simulink model "read_power_16chan"  (R2013a)
settings: Solver=VariableStepDiscrete  StartTime=0.0  StopTime=10000  RelTol=1e-3
libraries: xbsIndex_r4 x649, casper_library_misc x36, simulink x16, xps_library x1
(part 1 of 7)
settings Model: Creator=root  LastModifiedBy=root

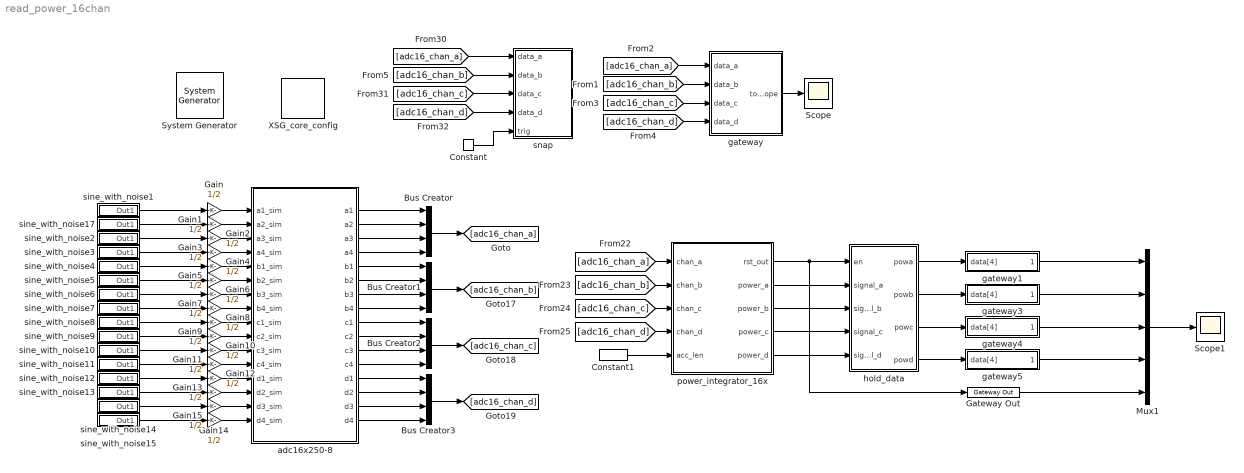
== system read_power_16chan ==
  " System Generator" : xbsIndex_r4/ System Generator  Tag=genX  xilinxfamily=virtex6  part=xc6vsx475t  speed=-1  package=ff1759  synthesis_tool=XST  clock_wrapper=Clock Enables  directory=./read_power_16chan/sysgen  proj_type=Project Navigator  Synth_file=XST Defaults  Impl_file=ISE Defaults  testbench=off  simulink_period=1  sysclk_period=5  dcm_input_clock_period=100  incr_netlist=off  trim_vbits=Everywhere in SubSystem  dbl_ovrd=According to Block Masks  core_generation=According to Block Masks  run_coregen=off  deprecated_control=off  eval_field=0  block_type=sysgen
  Bus Creator{,1..3} (4 alike) : BusCreator
  Constant : xbsIndex_r4/Constant  const=1  gui_display_data_type=Boolean  arith_type=Boolean  n_bits=16  bin_pt=14  preci_type=Single  exp_width=8  frac_width=24  explicit_period=off  period=1  equ=P=C  opselect=C  inp2=PCIN>>17  opr=+  inp1=P  carry=CIN  dbl_ovrd=off  block_type=constant
  Constant1 : xbsIndex_r4/Constant  const=255  gui_display_data_type=Fixed-point  arith_type=Unsigned  n_bits=10  bin_pt=0  preci_type=Single  exp_width=8  frac_width=24  explicit_period=off  period=1  equ=P=C  opselect=C  inp2=PCIN>>17  opr=+  inp1=P  carry=CIN  dbl_ovrd=off  block_type=constant
  Gain{,1..15} (16 alike) : Gain  Gain=1/2
  Gateway Out : xbsIndex_r4/Gateway Out  inherit_from_input=off  hdl_port=on  timing_constraint=None  locs_specified=off  LOCs={}  UseAsDAC=off  DACChannel='1'  block_type=gatewayout
  Mux1 : Mux  Inputs=5
  Scope : Scope
  Scope1 : Scope
  XSG_core_config : xps_library/XSG_core_config  Tag=xps:xsg  hw_sys=ROACH2:sx475t  clk_src=adc0_clk  ROACH_clk_src=sys_clk  ROACH2_clk_src=adc0_clk  MKDIG_clk_src=sys_clk  clk_rate=200  sample_period=1  synthesis_tool=XST
  adc16x250-8 : Subsystem  Tag=xps:adc16  AncestorBlock=xps_library/ADCs/adc16x250-8  mask(ADC16){board_count=1, roach2_rev=2, zdok_rev=2}
      mask prompts: board_count "Number of ADC16 Boards"; roach2_rev "ROACH2 Revision"; zdok_rev "ZDOK Pinout Revision"
      mask help: 16-input ADC. When using one ADC16 board, it must be in ZDOK0.
      mask init:
      | % Only board_count is needed by init function
      | adc16_init(gcb, ...
      |     'board_count', board_count);
      settings: AttributesFormatString=r2 rev%<roach2_rev>\nzdok rev%<zdok_rev>
      mask Help:
      | This is the CASPER "yellow block" for the CASPER ADC16 board.  Each ADC
      | board has four ADC chips.  Each ADC chip accepts four inputs.  The four
      | 8-bit outputs from each ADC chip are concatenated into a 32-bit signal.
      mask TypeOptions board_count: 1 | 2
      mask TypeOptions roach2_rev: 1 | 2
      mask TypeOptions zdok_rev: 1 | 2
  gateway : Subsystem
  gateway1 : Subsystem
  gateway3 : Subsystem
  gateway4 : Subsystem
  gateway5 : Subsystem
  hold_data : Subsystem
  power_integrator_16x : Subsystem
  sine_with_noise1 : Subsystem
  sine_with_noise10 : Subsystem
  sine_with_noise11 : Subsystem
  sine_with_noise12 : Subsystem
  sine_with_noise13 : Subsystem
  sine_with_noise14 : Subsystem
  sine_with_noise15 : Subsystem
  sine_with_noise17 : Subsystem
  sine_with_noise2 : Subsystem
  sine_with_noise3 : Subsystem
  sine_with_noise4 : Subsystem
  sine_with_noise5 : Subsystem
  sine_with_noise6 : Subsystem
  sine_with_noise7 : Subsystem
  sine_with_noise8 : Subsystem
  sine_with_noise9 : Subsystem
  snap : Subsystem
  wires:
  adc16x250-8/3(a3) -> Bus Creator/3
  adc16x250-8/2(a2) -> Bus Creator/2
  adc16x250-8/4(a4) -> Bus Creator/4
  Constant/1 -> snap/5(trig)
  gateway/1(to_scope) -> Scope/1
  adc16x250-8/1(a1) -> Bus Creator/1
  Bus Creator/1 -> [adc16_chan_a]
  power_integrator_16x/2(power_a) -> hold_data/2(signal_a)
  hold_data/1(powa) -> gateway1/1(data[4])
  power_integrator_16x/1(rst_out) -> Gateway Out/1, hold_data/1(en)
  Mux1/1 -> Scope1/1
  Gateway Out/1 -> Mux1/5
  [adc16_chan_a] -> gateway/1(data_a)
  Constant1/1 -> power_integrator_16x/5(acc_len)
  adc16x250-8/8(b4) -> Bus Creator1/4
  adc16x250-8/6(b2) -> Bus Creator1/2
  adc16x250-8/7(b3) -> Bus Creator1/3
  adc16x250-8/5(b1) -> Bus Creator1/1
  adc16x250-8/12(c4) -> Bus Creator2/4
  adc16x250-8/11(c3) -> Bus Creator2/3
  adc16x250-8/10(c2) -> Bus Creator2/2
  adc16x250-8/9(c1) -> Bus Creator2/1
  adc16x250-8/15(d3) -> Bus Creator3/3
  adc16x250-8/16(d4) -> Bus Creator3/4
  adc16x250-8/14(d2) -> Bus Creator3/2
  adc16x250-8/13(d1) -> Bus Creator3/1
  Bus Creator1/1 -> [adc16_chan_b]
  Bus Creator2/1 -> [adc16_chan_c]
  Bus Creator3/1 -> [adc16_chan_d]
  [adc16_chan_a] -> power_integrator_16x/1(chan_a)
  [adc16_chan_b] -> power_integrator_16x/2(chan_b)
  [adc16_chan_c] -> power_integrator_16x/3(chan_c)
  [adc16_chan_d] -> power_integrator_16x/4(chan_d)
  power_integrator_16x/3(power_b) -> hold_data/3(signal_b)
  power_integrator_16x/4(power_c) -> hold_data/4(signal_c)
  power_integrator_16x/5(power_d) -> hold_data/5(signal_d)
  hold_data/2(powb) -> gateway3/1(data[4])
  hold_data/3(powc) -> gateway4/1(data[4])
  hold_data/4(powd) -> gateway5/1(data[4])
  gateway1/1(to_scope) -> Mux1/1
  gateway3/1(to_scope) -> Mux1/2
  gateway4/1(to_scope) -> Mux1/3
  gateway5/1(to_scope) -> Mux1/4
  [adc16_chan_b] -> gateway/2(data_b)
  [adc16_chan_c] -> gateway/3(data_c)
  [adc16_chan_d] -> gateway/4(data_d)
  [adc16_chan_c] -> snap/3(data_c)
  [adc16_chan_b] -> snap/2(data_b)
  [adc16_chan_d] -> snap/4(data_d)
  [adc16_chan_a] -> snap/1(data_a)
  sine_with_noise1/1(Out1) -> Gain/1
  Gain/1 -> adc16x250-8/1(a1_sim)
  Gain1/1 -> adc16x250-8/2(a2_sim)
  Gain2/1 -> adc16x250-8/3(a3_sim)
  Gain3/1 -> adc16x250-8/4(a4_sim)
  Gain4/1 -> adc16x250-8/5(b1_sim)
  Gain5/1 -> adc16x250-8/6(b2_sim)
  Gain6/1 -> adc16x250-8/7(b3_sim)
  Gain7/1 -> adc16x250-8/8(b4_sim)
  Gain10/1 -> adc16x250-8/11(c3_sim)
  Gain8/1 -> adc16x250-8/9(c1_sim)
  Gain12/1 -> adc16x250-8/13(d1_sim)
  Gain15/1 -> adc16x250-8/16(d4_sim)
  Gain11/1 -> adc16x250-8/12(c4_sim)
  Gain14/1 -> adc16x250-8/15(d3_sim)
  Gain9/1 -> adc16x250-8/10(c2_sim)
  Gain13/1 -> adc16x250-8/14(d2_sim)
  sine_with_noise17/1(Out1) -> Gain1/1
  sine_with_noise2/1(Out1) -> Gain2/1
  sine_with_noise3/1(Out1) -> Gain3/1
  sine_with_noise4/1(Out1) -> Gain4/1
  sine_with_noise5/1(Out1) -> Gain5/1
  sine_with_noise6/1(Out1) -> Gain6/1
  sine_with_noise7/1(Out1) -> Gain7/1
  sine_with_noise8/1(Out1) -> Gain8/1
  sine_with_noise9/1(Out1) -> Gain9/1
  sine_with_noise10/1(Out1) -> Gain10/1
  sine_with_noise11/1(Out1) -> Gain11/1
  sine_with_noise12/1(Out1) -> Gain12/1
  sine_with_noise13/1(Out1) -> Gain13/1
  sine_with_noise14/1(Out1) -> Gain14/1
  sine_with_noise15/1(Out1) -> Gain15/1

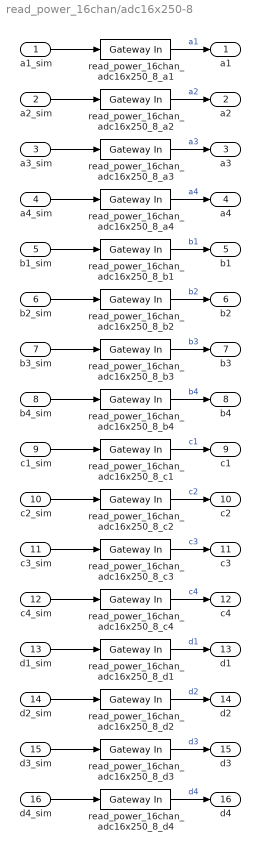
== system read_power_16chan/adc16x250-8 ==
  a1_sim : Inport
  a2_sim : Inport  Port=2
  a3_sim : Inport  Port=3
  a4_sim : Inport  Port=4
  b1_sim : Inport  Port=5
  b2_sim : Inport  Port=6
  b3_sim : Inport  Port=7
  b4_sim : Inport  Port=8
  c1_sim : Inport  Port=9
  c2_sim : Inport  Port=10
  c3_sim : Inport  Port=11
  c4_sim : Inport  Port=12
  d1_sim : Inport  Port=13
  d2_sim : Inport  Port=14
  d3_sim : Inport  Port=15
  d4_sim : Inport  Port=16
  read_power_16chan_adc16x250_8_a{1..4} (4 alike) : xbsIndex_r4/Gateway In  gui_display_data_type=Fixed-point  arith_type="Signed  (2's comp)"  n_bits=8  bin_pt=7  preci_type=Single  exp_width=8  frac_width=24  quantization="Round  (unbiased: +/- Inf)"  overflow=Saturate  period=1  dbl_ovrd=off  timing_constraint=None  locs_specified=off  LOCs={}  UseAsADC=off  ADCChannel='1'  inherit_from_input=off  hdl_port=on  block_type=gatewayin
  read_power_16chan_adc16x250_8_b{1..4} (4 alike) : xbsIndex_r4/Gateway In  gui_display_data_type=Fixed-point  arith_type="Signed  (2's comp)"  n_bits=8  bin_pt=7  preci_type=Single  exp_width=8  frac_width=24  quantization="Round  (unbiased: +/- Inf)"  overflow=Saturate  period=1  dbl_ovrd=off  timing_constraint=None  locs_specified=off  LOCs={}  UseAsADC=off  ADCChannel='1'  inherit_from_input=off  hdl_port=on  block_type=gatewayin
  read_power_16chan_adc16x250_8_c{1..4} (4 alike) : xbsIndex_r4/Gateway In  gui_display_data_type=Fixed-point  arith_type="Signed  (2's comp)"  n_bits=8  bin_pt=7  preci_type=Single  exp_width=8  frac_width=24  quantization="Round  (unbiased: +/- Inf)"  overflow=Saturate  period=1  dbl_ovrd=off  timing_constraint=None  locs_specified=off  LOCs={}  UseAsADC=off  ADCChannel='1'  inherit_from_input=off  hdl_port=on  block_type=gatewayin
  read_power_16chan_adc16x250_8_d{1..4} (4 alike) : xbsIndex_r4/Gateway In  gui_display_data_type=Fixed-point  arith_type="Signed  (2's comp)"  n_bits=8  bin_pt=7  preci_type=Single  exp_width=8  frac_width=24  quantization="Round  (unbiased: +/- Inf)"  overflow=Saturate  period=1  dbl_ovrd=off  timing_constraint=None  locs_specified=off  LOCs={}  UseAsADC=off  ADCChannel='1'  inherit_from_input=off  hdl_port=on  block_type=gatewayin
  a1 : Outport
  a2 : Outport  Port=2
  a3 : Outport  Port=3
  a4 : Outport  Port=4
  b1 : Outport  Port=5
  b2 : Outport  Port=6
  b3 : Outport  Port=7
  b4 : Outport  Port=8
  c1 : Outport  Port=9
  c2 : Outport  Port=10
  c3 : Outport  Port=11
  c4 : Outport  Port=12
  d1 : Outport  Port=13
  d2 : Outport  Port=14
  d3 : Outport  Port=15
  d4 : Outport  Port=16
  wires:
  a1_sim/1 -> read_power_16chan_adc16x250_8_a1/1
  read_power_16chan_adc16x250_8_a1/1 -> a1/1  "a1"
  a2_sim/1 -> read_power_16chan_adc16x250_8_a2/1
  read_power_16chan_adc16x250_8_a2/1 -> a2/1  "a2"
  a3_sim/1 -> read_power_16chan_adc16x250_8_a3/1
  read_power_16chan_adc16x250_8_a3/1 -> a3/1  "a3"
  a4_sim/1 -> read_power_16chan_adc16x250_8_a4/1
  read_power_16chan_adc16x250_8_a4/1 -> a4/1  "a4"
  b1_sim/1 -> read_power_16chan_adc16x250_8_b1/1
  read_power_16chan_adc16x250_8_b1/1 -> b1/1  "b1"
  b2_sim/1 -> read_power_16chan_adc16x250_8_b2/1
  read_power_16chan_adc16x250_8_b2/1 -> b2/1  "b2"
  b3_sim/1 -> read_power_16chan_adc16x250_8_b3/1
  read_power_16chan_adc16x250_8_b3/1 -> b3/1  "b3"
  b4_sim/1 -> read_power_16chan_adc16x250_8_b4/1
  read_power_16chan_adc16x250_8_b4/1 -> b4/1  "b4"
  c1_sim/1 -> read_power_16chan_adc16x250_8_c1/1
  read_power_16chan_adc16x250_8_c1/1 -> c1/1  "c1"
  c2_sim/1 -> read_power_16chan_adc16x250_8_c2/1
  read_power_16chan_adc16x250_8_c2/1 -> c2/1  "c2"
  c3_sim/1 -> read_power_16chan_adc16x250_8_c3/1
  read_power_16chan_adc16x250_8_c3/1 -> c3/1  "c3"
  c4_sim/1 -> read_power_16chan_adc16x250_8_c4/1
  read_power_16chan_adc16x250_8_c4/1 -> c4/1  "c4"
  d1_sim/1 -> read_power_16chan_adc16x250_8_d1/1
  read_power_16chan_adc16x250_8_d1/1 -> d1/1  "d1"
  d2_sim/1 -> read_power_16chan_adc16x250_8_d2/1
  read_power_16chan_adc16x250_8_d2/1 -> d2/1  "d2"
  d3_sim/1 -> read_power_16chan_adc16x250_8_d3/1
  read_power_16chan_adc16x250_8_d3/1 -> d3/1  "d3"
  d4_sim/1 -> read_power_16chan_adc16x250_8_d4/1
  read_power_16chan_adc16x250_8_d4/1 -> d4/1  "d4"

== system read_power_16chan/gateway ==
  data_a : Inport
  data_b : Inport  Port=2
  data_c : Inport  Port=3
  data_d : Inport  Port=4
  Bus Creator : BusCreator  Inputs=16
  Bus Selector : BusSelector  OutputSignals=a1,a2,a3,a4
  Bus Selector1 : BusSelector  OutputSignals=b1,b2,b3,b4
  Bus Selector2 : BusSelector  OutputSignals=c1,c2,c3,c4
  Bus Selector3 : BusSelector  OutputSignals=d1,d2,d3,d4
  Gateway Out{,1..15} (16 alike) : xbsIndex_r4/Gateway Out  inherit_from_input=off  hdl_port=on  timing_constraint=None  locs_specified=off  LOCs={}  UseAsDAC=off  DACChannel='1'  block_type=gatewayout
  to_scope : Outport
  wires:
  data_a/1 -> Bus Selector/1
  Bus Selector3/4 -> Gateway Out13/1  "<d4>"
  Bus Selector3/3 -> Gateway Out12/1  "<d3>"
  Bus Selector3/2 -> Gateway Out15/1  "<d2>"
  Bus Selector3/1 -> Gateway Out14/1  "<d1>"
  Bus Selector2/4 -> Gateway Out11/1  "<c4>"
  Bus Selector2/3 -> Gateway Out10/1  "<c3>"
  Bus Selector2/2 -> Gateway Out9/1  "<c2>"
  Bus Selector2/1 -> Gateway Out8/1  "<c1>"
  Bus Selector1/2 -> Gateway Out5/1  "<b2>"
  Bus Selector1/1 -> Gateway Out4/1  "<b1>"
  Bus Selector1/4 -> Gateway Out7/1  "<b4>"
  Bus Selector1/3 -> Gateway Out6/1  "<b3>"
  Bus Selector/4 -> Gateway Out3/1  "<a4>"
  Bus Selector/2 -> Gateway Out1/1  "<a2>"
  Bus Selector/1 -> Gateway Out/1  "<a1>"
  Bus Selector/3 -> Gateway Out2/1  "<a3>"
  Bus Creator/1 -> to_scope/1
  Gateway Out4/1 -> Bus Creator/5
  Gateway Out11/1 -> Bus Creator/12
  Gateway Out10/1 -> Bus Creator/11
  Gateway Out5/1 -> Bus Creator/6
  Gateway Out9/1 -> Bus Creator/10
  Gateway Out6/1 -> Bus Creator/7
  Gateway Out8/1 -> Bus Creator/9
  Gateway Out13/1 -> Bus Creator/16
  Gateway Out/1 -> Bus Creator/1
  Gateway Out7/1 -> Bus Creator/8
  Gateway Out1/1 -> Bus Creator/2
  Gateway Out12/1 -> Bus Creator/15
  Gateway Out15/1 -> Bus Creator/14
  Gateway Out2/1 -> Bus Creator/3
  Gateway Out3/1 -> Bus Creator/4
  Gateway Out14/1 -> Bus Creator/13
  data_b/1 -> Bus Selector1/1
  data_c/1 -> Bus Selector2/1
  data_d/1 -> Bus Selector3/1

== system read_power_16chan/gateway1 ==
  data[4] : Inport
  Bus Creator : BusCreator
  Bus Selector : BusSelector  OutputSignals=signal1,signal2,signal3,signal4
  Gateway Out{,1..3} (4 alike) : xbsIndex_r4/Gateway Out  inherit_from_input=off  hdl_port=on  timing_constraint=None  locs_specified=off  LOCs={}  UseAsDAC=off  DACChannel='1'  block_type=gatewayout
  to_scope : Outport
  wires:
  Gateway Out3/1 -> Bus Creator/4
  Gateway Out2/1 -> Bus Creator/3
  Gateway Out1/1 -> Bus Creator/2
  Gateway Out/1 -> Bus Creator/1
  Bus Creator/1 -> to_scope/1
  Bus Selector/3 -> Gateway Out2/1  "<signal3>"
  Bus Selector/1 -> Gateway Out/1  "<signal1>"
  Bus Selector/2 -> Gateway Out1/1  "<signal2>"
  Bus Selector/4 -> Gateway Out3/1  "<signal4>"
  data[4]/1 -> Bus Selector/1

== system read_power_16chan/gateway3 ==
  data[4] : Inport
  Bus Creator : BusCreator
  Bus Selector : BusSelector  OutputSignals=signal1,signal2,signal3,signal4
  Gateway Out{,1..3} (4 alike) : xbsIndex_r4/Gateway Out  inherit_from_input=off  hdl_port=on  timing_constraint=None  locs_specified=off  LOCs={}  UseAsDAC=off  DACChannel='1'  block_type=gatewayout
  to_scope : Outport
  wires:
  data[4]/1 -> Bus Selector/1
  Bus Selector/4 -> Gateway Out3/1  "<signal4>"
  Bus Selector/2 -> Gateway Out1/1  "<signal2>"
  Bus Selector/1 -> Gateway Out/1  "<signal1>"
  Bus Selector/3 -> Gateway Out2/1  "<signal3>"
  Bus Creator/1 -> to_scope/1
  Gateway Out/1 -> Bus Creator/1
  Gateway Out1/1 -> Bus Creator/2
  Gateway Out2/1 -> Bus Creator/3
  Gateway Out3/1 -> Bus Creator/4

== system read_power_16chan/gateway4 ==
  data[4] : Inport
  Bus Creator : BusCreator
  Bus Selector : BusSelector  OutputSignals=signal1,signal2,signal3,signal4
  Gateway Out{,1..3} (4 alike) : xbsIndex_r4/Gateway Out  inherit_from_input=off  hdl_port=on  timing_constraint=None  locs_specified=off  LOCs={}  UseAsDAC=off  DACChannel='1'  block_type=gatewayout
  to_scope : Outport
  wires:
  Gateway Out3/1 -> Bus Creator/4
  Gateway Out2/1 -> Bus Creator/3
  Gateway Out1/1 -> Bus Creator/2
  Gateway Out/1 -> Bus Creator/1
  Bus Creator/1 -> to_scope/1
  Bus Selector/3 -> Gateway Out2/1  "<signal3>"
  Bus Selector/1 -> Gateway Out/1  "<signal1>"
  Bus Selector/2 -> Gateway Out1/1  "<signal2>"
  Bus Selector/4 -> Gateway Out3/1  "<signal4>"
  data[4]/1 -> Bus Selector/1

== system read_power_16chan/gateway5 ==
  data[4] : Inport
  Bus Creator : BusCreator
  Bus Selector : BusSelector  OutputSignals=signal1,signal2,signal3,signal4
  Gateway Out{,1..3} (4 alike) : xbsIndex_r4/Gateway Out  inherit_from_input=off  hdl_port=on  timing_constraint=None  locs_specified=off  LOCs={}  UseAsDAC=off  DACChannel='1'  block_type=gatewayout
  to_scope : Outport
  wires:
  data[4]/1 -> Bus Selector/1
  Bus Selector/4 -> Gateway Out3/1  "<signal4>"
  Bus Selector/2 -> Gateway Out1/1  "<signal2>"
  Bus Selector/1 -> Gateway Out/1  "<signal1>"
  Bus Selector/3 -> Gateway Out2/1  "<signal3>"
  Bus Creator/1 -> to_scope/1
  Gateway Out/1 -> Bus Creator/1
  Gateway Out1/1 -> Bus Creator/2
  Gateway Out2/1 -> Bus Creator/3
  Gateway Out3/1 -> Bus Creator/4

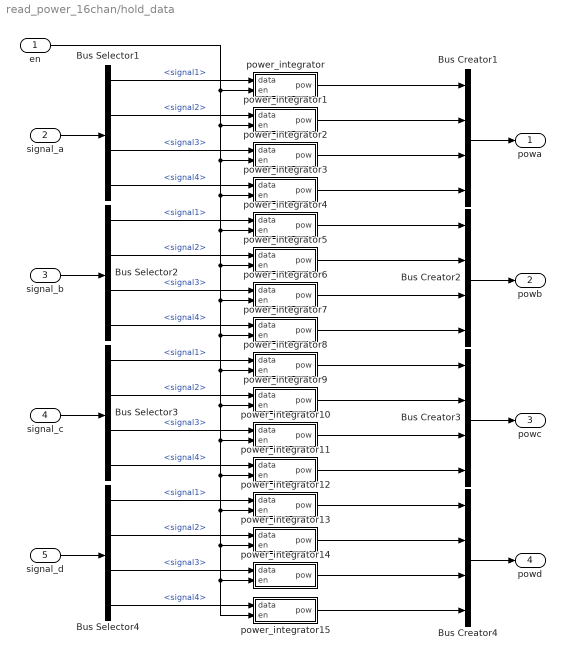
== system read_power_16chan/hold_data ==
  en : Inport
  signal_a : Inport  Port=2
  signal_b : Inport  Port=3
  signal_c : Inport  Port=4
  signal_d : Inport  Port=5
  Bus Creator{1..4} (4 alike) : BusCreator
  Bus Selector{1..4} (4 alike) : BusSelector  OutputSignals=signal1,signal2,signal3,signal4
  power_integrator : Subsystem
  power_integrator1 : Subsystem
  power_integrator10 : Subsystem
  power_integrator11 : Subsystem
  power_integrator12 : Subsystem
  power_integrator13 : Subsystem
  power_integrator14 : Subsystem
  power_integrator15 : Subsystem
  power_integrator2 : Subsystem
  power_integrator3 : Subsystem
  power_integrator4 : Subsystem
  power_integrator5 : Subsystem
  power_integrator6 : Subsystem
  power_integrator7 : Subsystem
  power_integrator8 : Subsystem
  power_integrator9 : Subsystem
  powa : Outport
  powb : Outport  Port=2
  powc : Outport  Port=3
  powd : Outport  Port=4
  wires:
  power_integrator4/1(pow) -> Bus Creator2/1
  power_integrator1/1(pow) -> Bus Creator1/2
  power_integrator5/1(pow) -> Bus Creator2/2
  power_integrator6/1(pow) -> Bus Creator2/3
  power_integrator2/1(pow) -> Bus Creator1/3
  power_integrator7/1(pow) -> Bus Creator2/4
  power_integrator3/1(pow) -> Bus Creator1/4
  Bus Creator1/1 -> powa/1
  power_integrator/1(pow) -> Bus Creator1/1
  power_integrator11/1(pow) -> Bus Creator3/4
  power_integrator8/1(pow) -> Bus Creator3/1
  power_integrator14/1(pow) -> Bus Creator4/3
  power_integrator12/1(pow) -> Bus Creator4/1
  power_integrator15/1(pow) -> Bus Creator4/4
  power_integrator10/1(pow) -> Bus Creator3/3
  power_integrator9/1(pow) -> Bus Creator3/2
  power_integrator13/1(pow) -> Bus Creator4/2
  en/1 -> power_integrator15/2(en), power_integrator14/2(en), power_integrator13/2(en), power_integrator12/2(en), power_integrator11/2(en), power_integrator10/2(en), power_integrator9/2(en), power_integrator8/2(en), power_integrator7/2(en), power_integrator6/2(en), power_integrator5/2(en), power_integrator4/2(en), power_integrator3/2(en), power_integrator2/2(en), power_integrator1/2(en), power_integrator/2(en)
  signal_a/1 -> Bus Selector1/1
  signal_d/1 -> Bus Selector4/1
  signal_c/1 -> Bus Selector3/1
  Bus Selector1/1 -> power_integrator/1(data)  "<signal1>"
  Bus Selector1/2 -> power_integrator1/1(data)  "<signal2>"
  Bus Selector1/3 -> power_integrator2/1(data)  "<signal3>"
  Bus Selector1/4 -> power_integrator3/1(data)  "<signal4>"
  signal_b/1 -> Bus Selector2/1
  Bus Selector2/1 -> power_integrator4/1(data)  "<signal1>"
  Bus Selector2/2 -> power_integrator5/1(data)  "<signal2>"
  Bus Selector2/3 -> power_integrator6/1(data)  "<signal3>"
  Bus Selector2/4 -> power_integrator7/1(data)  "<signal4>"
  Bus Selector3/1 -> power_integrator8/1(data)  "<signal1>"
  Bus Selector3/2 -> power_integrator9/1(data)  "<signal2>"
  Bus Selector3/3 -> power_integrator10/1(data)  "<signal3>"
  Bus Selector3/4 -> power_integrator11/1(data)  "<signal4>"
  Bus Selector4/1 -> power_integrator12/1(data)  "<signal1>"
  Bus Selector4/2 -> power_integrator13/1(data)  "<signal2>"
  Bus Selector4/3 -> power_integrator14/1(data)  "<signal3>"
  Bus Selector4/4 -> power_integrator15/1(data)  "<signal4>"
  Bus Creator4/1 -> powd/1
  Bus Creator3/1 -> powc/1
  Bus Creator2/1 -> powb/1

== system read_power_16chan/power_integrator_16x ==
  chan_a : Inport
  chan_b : Inport  Port=2
  chan_c : Inport  Port=3
  chan_d : Inport  Port=4
  acc_len : Inport  Port=5
  Bus Creator{,1..3} (4 alike) : BusCreator
  Bus Selector : BusSelector  OutputSignals=a1,a2,a3,a4
  Bus Selector1 : BusSelector  OutputSignals=b1,b2,b3,b4
  Bus Selector2 : BusSelector  OutputSignals=c1,c2,c3,c4
  Bus Selector3 : BusSelector  OutputSignals=d1,d2,d3,d4
  Terminator : Terminator
  Terminator1 : Terminator
  Terminator2 : Terminator
  power_integrator_4x : Subsystem
  power_integrator_4x1 : Subsystem
  power_integrator_4x2 : Subsystem
  power_integrator_4x3 : Subsystem
  rst_out : Outport
  power_a : Outport  Port=2
  power_b : Outport  Port=3
  power_c : Outport  Port=4
  power_d : Outport  Port=5
  wires:
  power_integrator_4x/1(rst) -> rst_out/1
  acc_len/1 -> power_integrator_4x3/5(acc_len), power_integrator_4x2/5(acc_len), power_integrator_4x1/5(acc_len), power_integrator_4x/5(acc_len)
  Bus Selector/4 -> power_integrator_4x/4(in4)  "<a4>"
  Bus Selector/2 -> power_integrator_4x/2(in2)  "<a2>"
  Bus Selector/3 -> power_integrator_4x/3(in3)  "<a3>"
  Bus Selector/1 -> power_integrator_4x/1(in1)  "<a1>"
  chan_a/1 -> Bus Selector/1
  Bus Selector1/4 -> power_integrator_4x1/4(in4)  "<b4>"
  Bus Selector1/1 -> power_integrator_4x1/1(in1)  "<b1>"
  Bus Selector1/3 -> power_integrator_4x1/3(in3)  "<b3>"
  Bus Selector1/2 -> power_integrator_4x1/2(in2)  "<b2>"
  chan_b/1 -> Bus Selector1/1
  chan_d/1 -> Bus Selector3/1
  chan_c/1 -> Bus Selector2/1
  Bus Selector2/2 -> power_integrator_4x2/2(in2)  "<c2>"
  Bus Selector2/3 -> power_integrator_4x2/3(in3)  "<c3>"
  Bus Selector2/1 -> power_integrator_4x2/1(in1)  "<c1>"
  Bus Selector2/4 -> power_integrator_4x2/4(in4)  "<c4>"
  Bus Selector3/3 -> power_integrator_4x3/3(in3)  "<d3>"
  Bus Selector3/1 -> power_integrator_4x3/1(in1)  "<d1>"
  Bus Selector3/2 -> power_integrator_4x3/2(in2)  "<d2>"
  Bus Selector3/4 -> power_integrator_4x3/4(in4)  "<d4>"
  power_integrator_4x1/1(rst) -> Terminator/1
  power_integrator_4x2/1(rst) -> Terminator1/1
  power_integrator_4x3/1(rst) -> Terminator2/1
  power_integrator_4x/3(pow2) -> Bus Creator/2
  power_integrator_4x/5(pow4) -> Bus Creator/4
  power_integrator_4x/4(pow3) -> Bus Creator/3
  power_integrator_4x/2(pow1) -> Bus Creator/1
  Bus Creator/1 -> power_a/1
  power_integrator_4x1/3(pow2) -> Bus Creator1/2
  power_integrator_4x1/2(pow1) -> Bus Creator1/1
  power_integrator_4x1/5(pow4) -> Bus Creator1/4
  power_integrator_4x1/4(pow3) -> Bus Creator1/3
  Bus Creator1/1 -> power_b/1
  power_integrator_4x2/5(pow4) -> Bus Creator2/4
  power_integrator_4x2/4(pow3) -> Bus Creator2/3
  power_integrator_4x2/3(pow2) -> Bus Creator2/2
  power_integrator_4x2/2(pow1) -> Bus Creator2/1
  Bus Creator2/1 -> power_c/1
  power_integrator_4x3/5(pow4) -> Bus Creator3/4
  power_integrator_4x3/2(pow1) -> Bus Creator3/1
  power_integrator_4x3/4(pow3) -> Bus Creator3/3
  power_integrator_4x3/3(pow2) -> Bus Creator3/2
  Bus Creator3/1 -> power_d/1

== system read_power_16chan/sine_with_noise1 ==
  Add : Sum
  Band-Limited White Noise : simulink/Sources/Band-Limited White Noise  Cov=[0.001]  Ts=1  seed=[232]
  Sine Wave : Sin  SineType=Sample based  Samples=25  SampleTime=1
  Out1 : Outport
  wires:
  Sine Wave/1 -> Add/1
  Add/1 -> Out1/1
  Band-Limited White Noise/1 -> Add/2

== system read_power_16chan/sine_with_noise10 ==
  Add : Sum
  Band-Limited White Noise : simulink/Sources/Band-Limited White Noise  Cov=[0.001]  Ts=1  seed=[232]
  Sine Wave : Sin  SineType=Sample based  Samples=25  SampleTime=1
  Out1 : Outport
  wires:
  Sine Wave/1 -> Add/1
  Add/1 -> Out1/1
  Band-Limited White Noise/1 -> Add/2

== system read_power_16chan/sine_with_noise11 ==
  Add : Sum
  Band-Limited White Noise : simulink/Sources/Band-Limited White Noise  Cov=[0.001]  Ts=1  seed=[232]
  Sine Wave : Sin  SineType=Sample based  Samples=25  SampleTime=1
  Out1 : Outport
  wires:
  Band-Limited White Noise/1 -> Add/2
  Add/1 -> Out1/1
  Sine Wave/1 -> Add/1

== system read_power_16chan/sine_with_noise12 ==
  Add : Sum
  Band-Limited White Noise : simulink/Sources/Band-Limited White Noise  Cov=[0.001]  Ts=1  seed=[232]
  Sine Wave : Sin  SineType=Sample based  Samples=25  SampleTime=1
  Out1 : Outport
  wires:
  Sine Wave/1 -> Add/1
  Add/1 -> Out1/1
  Band-Limited White Noise/1 -> Add/2

== system read_power_16chan/sine_with_noise13 ==
  Add : Sum
  Band-Limited White Noise : simulink/Sources/Band-Limited White Noise  Cov=[0.001]  Ts=1  seed=[232]
  Sine Wave : Sin  SineType=Sample based  Samples=25  SampleTime=1
  Out1 : Outport
  wires:
  Band-Limited White Noise/1 -> Add/2
  Add/1 -> Out1/1
  Sine Wave/1 -> Add/1

== system read_power_16chan/sine_with_noise14 ==
  Add : Sum
  Band-Limited White Noise : simulink/Sources/Band-Limited White Noise  Cov=[0.001]  Ts=1  seed=[232]
  Sine Wave : Sin  SineType=Sample based  Samples=25  SampleTime=1
  Out1 : Outport
  wires:
  Band-Limited White Noise/1 -> Add/2
  Add/1 -> Out1/1
  Sine Wave/1 -> Add/1

== system read_power_16chan/sine_with_noise15 ==
  Add : Sum
  Band-Limited White Noise : simulink/Sources/Band-Limited White Noise  Cov=[0.001]  Ts=1  seed=[232]
  Sine Wave : Sin  SineType=Sample based  Samples=25  SampleTime=1
  Out1 : Outport
  wires:
  Sine Wave/1 -> Add/1
  Add/1 -> Out1/1
  Band-Limited White Noise/1 -> Add/2

== system read_power_16chan/sine_with_noise17 ==
  Add : Sum
  Band-Limited White Noise : simulink/Sources/Band-Limited White Noise  Cov=[0.001]  Ts=1  seed=[232]
  Sine Wave : Sin  SineType=Sample based  Samples=25  SampleTime=1
  Out1 : Outport
  wires:
  Band-Limited White Noise/1 -> Add/2
  Add/1 -> Out1/1
  Sine Wave/1 -> Add/1

== system read_power_16chan/sine_with_noise2 ==
  Add : Sum
  Band-Limited White Noise : simulink/Sources/Band-Limited White Noise  Cov=[0.001]  Ts=1  seed=[232]
  Sine Wave : Sin  SineType=Sample based  Samples=25  SampleTime=1
  Out1 : Outport
  wires:
  Band-Limited White Noise/1 -> Add/2
  Add/1 -> Out1/1
  Sine Wave/1 -> Add/1

== system read_power_16chan/sine_with_noise3 ==
  Add : Sum
  Band-Limited White Noise : simulink/Sources/Band-Limited White Noise  Cov=[0.001]  Ts=1  seed=[232]
  Sine Wave : Sin  SineType=Sample based  Samples=25  SampleTime=1
  Out1 : Outport
  wires:
  Sine Wave/1 -> Add/1
  Add/1 -> Out1/1
  Band-Limited White Noise/1 -> Add/2

== system read_power_16chan/sine_with_noise4 ==
  Add : Sum
  Band-Limited White Noise : simulink/Sources/Band-Limited White Noise  Cov=[0.001]  Ts=1  seed=[232]
  Sine Wave : Sin  SineType=Sample based  Samples=25  SampleTime=1
  Out1 : Outport
  wires:
  Band-Limited White Noise/1 -> Add/2
  Add/1 -> Out1/1
  Sine Wave/1 -> Add/1

== system read_power_16chan/sine_with_noise5 ==
  Add : Sum
  Band-Limited White Noise : simulink/Sources/Band-Limited White Noise  Cov=[0.001]  Ts=1  seed=[232]
  Sine Wave : Sin  SineType=Sample based  Samples=25  SampleTime=1
  Out1 : Outport
  wires:
  Sine Wave/1 -> Add/1
  Add/1 -> Out1/1
  Band-Limited White Noise/1 -> Add/2

== system read_power_16chan/sine_with_noise6 ==
  Add : Sum
  Band-Limited White Noise : simulink/Sources/Band-Limited White Noise  Cov=[0.001]  Ts=1  seed=[232]
  Sine Wave : Sin  SineType=Sample based  Samples=25  SampleTime=1
  Out1 : Outport
  wires:
  Sine Wave/1 -> Add/1
  Add/1 -> Out1/1
  Band-Limited White Noise/1 -> Add/2

== system read_power_16chan/sine_with_noise7 ==
  Add : Sum
  Band-Limited White Noise : simulink/Sources/Band-Limited White Noise  Cov=[0.001]  Ts=1  seed=[232]
  Sine Wave : Sin  SineType=Sample based  Samples=25  SampleTime=1
  Out1 : Outport
  wires:
  Band-Limited White Noise/1 -> Add/2
  Add/1 -> Out1/1
  Sine Wave/1 -> Add/1

== system read_power_16chan/sine_with_noise8 ==
  Add : Sum
  Band-Limited White Noise : simulink/Sources/Band-Limited White Noise  Cov=[0.001]  Ts=1  seed=[232]
  Sine Wave : Sin  SineType=Sample based  Samples=25  SampleTime=1
  Out1 : Outport
  wires:
  Band-Limited White Noise/1 -> Add/2
  Add/1 -> Out1/1
  Sine Wave/1 -> Add/1

== system read_power_16chan/sine_with_noise9 ==
  Add : Sum
  Band-Limited White Noise : simulink/Sources/Band-Limited White Noise  Cov=[0.001]  Ts=1  seed=[232]
  Sine Wave : Sin  SineType=Sample based  Samples=25  SampleTime=1
  Out1 : Outport
  wires:
  Sine Wave/1 -> Add/1
  Add/1 -> Out1/1
  Band-Limited White Noise/1 -> Add/2

== system read_power_16chan/snap ==
  data_a : Inport
  data_b : Inport  Port=2
  data_c : Inport  Port=3
  data_d : Inport  Port=4
  trig : Inport  Port=5
  Bus Selector : BusSelector  OutputSignals=a1,a2,a3,a4
  Bus Selector1 : BusSelector  OutputSignals=b1,b2,b3,b4
  Bus Selector2 : BusSelector  OutputSignals=c1,c2,c3,c4
  Bus Selector3 : BusSelector  OutputSignals=d1,d2,d3,d4
  Constant : xbsIndex_r4/Constant  const=0  gui_display_data_type=Boolean  arith_type=Boolean  n_bits=16  bin_pt=14  preci_type=Single  exp_width=8  frac_width=24  explicit_period=off  period=1  equ=P=C  opselect=C  inp2=PCIN>>17  opr=+  inp1=P  carry=CIN  dbl_ovrd=off  block_type=constant
  a : Subsystem  Tag=casper:snapshot  AncestorBlock=casper_library_scopes/snapshot  mask(snapshot){storage=bram, dram_dimm=1, dram_clock=200, nsamples=16, data_width=32, offset=off, circap=off, value=off, use_dsp48=on}
      mask prompts: storage "Storage medium"; dram_dimm "DRAM dimm"; dram_clock "DRAM clock rate"; nsamples "Number of Samples (2^?)"; data_width "Data width"; offset "Start delay support"; circap "Circular capture support"; value "Extra value capture support"; use_dsp48 "Use DSP48s to implement counters"
      mask help:
      | Standard snap block, but with the following optional extras;
      |  1) Optionally delay the fabric trigger by a user-specified number of valids.
      |  2) Capture continuously after a trigger until a stop pulse is received. Data is captured into BRAM continuously, with old data being overwritten until a stop command is received. Then stop capturing when memory is filled. This enables you to get some data before and some data after the stop pulse. Use the 'tr_en_cnt' register to determine where you are in your vector. 'Addr' register's MSb now indicates 'busy capturing'.
      |  3) Optionally capture a value on an input port to a register at the same time as the first data sample.
      |  4) Implement counters using DSP48Es to save resources.
      mask init:
      | snapshot_init(gcb, ...
      |     'storage', storage, ...
      |     'dram_dimm', dram_dimm, ...
      |     'dram_clock', dram_clock, ...
      |     'nsamples', nsamples, ...
      |     'data_width', data_width, ...
      |     'offset', offset, ...
      |     'circap', circap, ...
      |     'value', value, ...
      |     'use_dsp48', use_dsp48);
      mask TypeOptions storage: bram | dram
      mask Callback storage: snapshot_callback();
      mask TypeOptions dram_dimm: 1 | 2 | 3 | 4
      mask TypeOptions dram_clock: 200 | 250 | 266 | 300 | 333
      mask TypeOptions data_width: 8 | 16 | 32 | 64 | 128
  b : Subsystem  Tag=casper:snapshot  AncestorBlock=casper_library_scopes/snapshot  mask(snapshot){storage=bram, dram_dimm=1, dram_clock=200, nsamples=16, data_width=32, offset=off, circap=off, value=off, use_dsp48=on}
      mask prompts: storage "Storage medium"; dram_dimm "DRAM dimm"; dram_clock "DRAM clock rate"; nsamples "Number of Samples (2^?)"; data_width "Data width"; offset "Start delay support"; circap "Circular capture support"; value "Extra value capture support"; use_dsp48 "Use DSP48s to implement counters"
      mask help:
      | Standard snap block, but with the following optional extras;
      |  1) Optionally delay the fabric trigger by a user-specified number of valids.
      |  2) Capture continuously after a trigger until a stop pulse is received. Data is captured into BRAM continuously, with old data being overwritten until a stop command is received. Then stop capturing when memory is filled. This enables you to get some data before and some data after the stop pulse. Use the 'tr_en_cnt' register to determine where you are in your vector. 'Addr' register's MSb now indicates 'busy capturing'.
      |  3) Optionally capture a value on an input port to a register at the same time as the first data sample.
      |  4) Implement counters using DSP48Es to save resources.
      mask init: same as read_power_16chan/snap/a
      mask TypeOptions storage: bram | dram
      mask Callback storage: snapshot_callback();
      mask TypeOptions dram_dimm: 1 | 2 | 3 | 4
      mask TypeOptions dram_clock: 200 | 250 | 266 | 300 | 333
      mask TypeOptions data_width: 8 | 16 | 32 | 64 | 128
  bus_create : Subsystem  AncestorBlock=casper_library_flow_control/bus_create  mask(bus_create){inputNum=4}
      mask prompts: inputNum "Number of inputs:"
      mask init:
      | bus_create_init(gcb,...
      |     'inputNum', inputNum);
  bus_create1 : Subsystem  AncestorBlock=casper_library_flow_control/bus_create  mask(bus_create){inputNum=4}
      mask prompts: inputNum "Number of inputs:"
      mask init:
      | bus_create_init(gcb,...
      |     'inputNum', inputNum);
  bus_create2 : Subsystem  AncestorBlock=casper_library_flow_control/bus_create  mask(bus_create){inputNum=4}
      mask prompts: inputNum "Number of inputs:"
      mask init:
      | bus_create_init(gcb,...
      |     'inputNum', inputNum);
  bus_create3 : Subsystem  AncestorBlock=casper_library_flow_control/bus_create  mask(bus_create){inputNum=4}
      mask prompts: inputNum "Number of inputs:"
      mask init:
      | bus_create_init(gcb,...
      |     'inputNum', inputNum);
  c : Subsystem  Tag=casper:snapshot  AncestorBlock=casper_library_scopes/snapshot  mask(snapshot){storage=bram, dram_dimm=1, dram_clock=200, nsamples=16, data_width=32, offset=off, circap=off, value=off, use_dsp48=on}
      mask prompts: storage "Storage medium"; dram_dimm "DRAM dimm"; dram_clock "DRAM clock rate"; nsamples "Number of Samples (2^?)"; data_width "Data width"; offset "Start delay support"; circap "Circular capture support"; value "Extra value capture support"; use_dsp48 "Use DSP48s to implement counters"
      mask help:
      | Standard snap block, but with the following optional extras;
      |  1) Optionally delay the fabric trigger by a user-specified number of valids.
      |  2) Capture continuously after a trigger until a stop pulse is received. Data is captured into BRAM continuously, with old data being overwritten until a stop command is received. Then stop capturing when memory is filled. This enables you to get some data before and some data after the stop pulse. Use the 'tr_en_cnt' register to determine where you are in your vector. 'Addr' register's MSb now indicates 'busy capturing'.
      |  3) Optionally capture a value on an input port to a register at the same time as the first data sample.
      |  4) Implement counters using DSP48Es to save resources.
      mask init: same as read_power_16chan/snap/a
      mask TypeOptions storage: bram | dram
      mask Callback storage: snapshot_callback();
      mask TypeOptions dram_dimm: 1 | 2 | 3 | 4
      mask TypeOptions dram_clock: 200 | 250 | 266 | 300 | 333
      mask TypeOptions data_width: 8 | 16 | 32 | 64 | 128
  d : Subsystem  Tag=casper:snapshot  AncestorBlock=casper_library_scopes/snapshot  mask(snapshot){storage=bram, dram_dimm=1, dram_clock=200, nsamples=16, data_width=32, offset=off, circap=off, value=off, use_dsp48=on}
      mask prompts: storage "Storage medium"; dram_dimm "DRAM dimm"; dram_clock "DRAM clock rate"; nsamples "Number of Samples (2^?)"; data_width "Data width"; offset "Start delay support"; circap "Circular capture support"; value "Extra value capture support"; use_dsp48 "Use DSP48s to implement counters"
      mask help:
      | Standard snap block, but with the following optional extras;
      |  1) Optionally delay the fabric trigger by a user-specified number of valids.
      |  2) Capture continuously after a trigger until a stop pulse is received. Data is captured into BRAM continuously, with old data being overwritten until a stop command is received. Then stop capturing when memory is filled. This enables you to get some data before and some data after the stop pulse. Use the 'tr_en_cnt' register to determine where you are in your vector. 'Addr' register's MSb now indicates 'busy capturing'.
      |  3) Optionally capture a value on an input port to a register at the same time as the first data sample.
      |  4) Implement counters using DSP48Es to save resources.
      mask init: same as read_power_16chan/snap/a
      mask TypeOptions storage: bram | dram
      mask Callback storage: snapshot_callback();
      mask TypeOptions dram_dimm: 1 | 2 | 3 | 4
      mask TypeOptions dram_clock: 200 | 250 | 266 | 300 | 333
      mask TypeOptions data_width: 8 | 16 | 32 | 64 | 128
  wires:
  Constant/1 -> d/2(we), c/2(we), b/2(we), a/2(we)
  trig/1 -> a/3(trig), b/3(trig), c/3(trig), d/3(trig)
  Bus Selector/3 -> bus_create/3(in3)  "<a3>"
  Bus Selector/1 -> bus_create/1(in1)  "<a1>"
  Bus Selector/2 -> bus_create/2(in2)  "<a2>"
  Bus Selector/4 -> bus_create/4(in4)  "<a4>"
  bus_create/1(bus_out) -> a/1(din)
  Bus Selector1/3 -> bus_create1/3(in3)  "<b3>"
  Bus Selector1/4 -> bus_create1/4(in4)  "<b4>"
  Bus Selector1/1 -> bus_create1/1(in1)  "<b1>"
  Bus Selector1/2 -> bus_create1/2(in2)  "<b2>"
  Bus Selector2/1 -> bus_create2/1(in1)  "<c1>"
  Bus Selector2/2 -> bus_create2/2(in2)  "<c2>"
  Bus Selector2/3 -> bus_create2/3(in3)  "<c3>"
  Bus Selector2/4 -> bus_create2/4(in4)  "<c4>"
  Bus Selector3/1 -> bus_create3/1(in1)  "<d1>"
  Bus Selector3/2 -> bus_create3/2(in2)  "<d2>"
  Bus Selector3/3 -> bus_create3/3(in3)  "<d3>"
  Bus Selector3/4 -> bus_create3/4(in4)  "<d4>"
  bus_create3/1(bus_out) -> d/1(din)
  bus_create2/1(bus_out) -> c/1(din)
  bus_create1/1(bus_out) -> b/1(din)
  data_a/1 -> Bus Selector/1
  data_d/1 -> Bus Selector3/1
  data_c/1 -> Bus Selector2/1
  data_b/1 -> Bus Selector1/1

== system read_power_16chan/hold_data/power_integrator ==
  data : Inport
  en : Inport  Port=2
  Register : xbsIndex_r4/Register  init=0  rst=off  en=on  dbl_ovrd=off  block_type=register
  pow : Outport
  wires:
  data/1 -> Register/1
  Register/1 -> pow/1
  en/1 -> Register/2

== system read_power_16chan/hold_data/power_integrator1 ==
  data : Inport
  en : Inport  Port=2
  Register : xbsIndex_r4/Register  init=0  rst=off  en=on  dbl_ovrd=off  block_type=register
  pow : Outport
  wires:
  en/1 -> Register/2
  Register/1 -> pow/1
  data/1 -> Register/1

== system read_power_16chan/hold_data/power_integrator10 ==
  data : Inport
  en : Inport  Port=2
  Register : xbsIndex_r4/Register  init=0  rst=off  en=on  dbl_ovrd=off  block_type=register
  pow : Outport
  wires:
  en/1 -> Register/2
  Register/1 -> pow/1
  data/1 -> Register/1

== system read_power_16chan/hold_data/power_integrator11 ==
  data : Inport
  en : Inport  Port=2
  Register : xbsIndex_r4/Register  init=0  rst=off  en=on  dbl_ovrd=off  block_type=register
  pow : Outport
  wires:
  data/1 -> Register/1
  Register/1 -> pow/1
  en/1 -> Register/2

== system read_power_16chan/hold_data/power_integrator12 ==
  data : Inport
  en : Inport  Port=2
  Register : xbsIndex_r4/Register  init=0  rst=off  en=on  dbl_ovrd=off  block_type=register
  pow : Outport
  wires:
  en/1 -> Register/2
  Register/1 -> pow/1
  data/1 -> Register/1

== system read_power_16chan/hold_data/power_integrator13 ==
  data : Inport
  en : Inport  Port=2
  Register : xbsIndex_r4/Register  init=0  rst=off  en=on  dbl_ovrd=off  block_type=register
  pow : Outport
  wires:
  data/1 -> Register/1
  Register/1 -> pow/1
  en/1 -> Register/2

== system read_power_16chan/hold_data/power_integrator14 ==
  data : Inport
  en : Inport  Port=2
  Register : xbsIndex_r4/Register  init=0  rst=off  en=on  dbl_ovrd=off  block_type=register
  pow : Outport
  wires:
  en/1 -> Register/2
  Register/1 -> pow/1
  data/1 -> Register/1

== system read_power_16chan/hold_data/power_integrator15 ==
  data : Inport
  en : Inport  Port=2
  Register : xbsIndex_r4/Register  init=0  rst=off  en=on  dbl_ovrd=off  block_type=register
  pow : Outport
  wires:
  data/1 -> Register/1
  Register/1 -> pow/1
  en/1 -> Register/2

== system read_power_16chan/hold_data/power_integrator2 ==
  data : Inport
  en : Inport  Port=2
  Register : xbsIndex_r4/Register  init=0  rst=off  en=on  dbl_ovrd=off  block_type=register
  pow : Outport
  wires:
  data/1 -> Register/1
  Register/1 -> pow/1
  en/1 -> Register/2

== system read_power_16chan/hold_data/power_integrator3 ==
  data : Inport
  en : Inport  Port=2
  Register : xbsIndex_r4/Register  init=0  rst=off  en=on  dbl_ovrd=off  block_type=register
  pow : Outport
  wires:
  en/1 -> Register/2
  Register/1 -> pow/1
  data/1 -> Register/1

== system read_power_16chan/hold_data/power_integrator4 ==
  data : Inport
  en : Inport  Port=2
  Register : xbsIndex_r4/Register  init=0  rst=off  en=on  dbl_ovrd=off  block_type=register
  pow : Outport
  wires:
  data/1 -> Register/1
  Register/1 -> pow/1
  en/1 -> Register/2

== system read_power_16chan/hold_data/power_integrator5 ==
  data : Inport
  en : Inport  Port=2
  Register : xbsIndex_r4/Register  init=0  rst=off  en=on  dbl_ovrd=off  block_type=register
  pow : Outport
  wires:
  en/1 -> Register/2
  Register/1 -> pow/1
  data/1 -> Register/1

== system read_power_16chan/hold_data/power_integrator6 ==
  data : Inport
  en : Inport  Port=2
  Register : xbsIndex_r4/Register  init=0  rst=off  en=on  dbl_ovrd=off  block_type=register
  pow : Outport
  wires:
  data/1 -> Register/1
  Register/1 -> pow/1
  en/1 -> Register/2

== system read_power_16chan/hold_data/power_integrator7 ==
  data : Inport
  en : Inport  Port=2
  Register : xbsIndex_r4/Register  init=0  rst=off  en=on  dbl_ovrd=off  block_type=register
  pow : Outport
  wires:
  en/1 -> Register/2
  Register/1 -> pow/1
  data/1 -> Register/1

== system read_power_16chan/hold_data/power_integrator8 ==
  data : Inport
  en : Inport  Port=2
  Register : xbsIndex_r4/Register  init=0  rst=off  en=on  dbl_ovrd=off  block_type=register
  pow : Outport
  wires:
  en/1 -> Register/2
  Register/1 -> pow/1
  data/1 -> Register/1

== system read_power_16chan/hold_data/power_integrator9 ==
  data : Inport
  en : Inport  Port=2
  Register : xbsIndex_r4/Register  init=0  rst=off  en=on  dbl_ovrd=off  block_type=register
  pow : Outport
  wires:
  data/1 -> Register/1
  Register/1 -> pow/1
  en/1 -> Register/2

== system read_power_16chan/power_integrator_16x/power_integrator_4x ==
  in1 : Inport
  in2 : Inport  Port=2
  in3 : Inport  Port=3
  in4 : Inport  Port=4
  acc_len : Inport  Port=5
  Terminator : Terminator
  Terminator1 : Terminator
  Terminator2 : Terminator
  power_integrator : Subsystem
  power_integrator1 : Subsystem
  power_integrator2 : Subsystem
  power_integrator3 : Subsystem
  rst : Outport
  pow1 : Outport  Port=2
  pow2 : Outport  Port=3
  pow3 : Outport  Port=4
  pow4 : Outport  Port=5
  wires:
  power_integrator1/2(rst_out) -> Terminator/1
  power_integrator2/2(rst_out) -> Terminator1/1
  power_integrator3/2(rst_out) -> Terminator2/1
  power_integrator/1(pow) -> pow1/1
  in1/1 -> power_integrator/1(signal)
  in2/1 -> power_integrator1/1(signal)
  in3/1 -> power_integrator2/1(signal)
  in4/1 -> power_integrator3/1(signal)
  power_integrator3/1(pow) -> pow4/1
  power_integrator2/1(pow) -> pow3/1
  power_integrator1/1(pow) -> pow2/1
  power_integrator/2(rst_out) -> rst/1
  acc_len/1 -> power_integrator3/2(acc_len), power_integrator2/2(acc_len), power_integrator1/2(acc_len), power_integrator/2(acc_len)

== system read_power_16chan/power_integrator_16x/power_integrator_4x1 ==
  in1 : Inport
  in2 : Inport  Port=2
  in3 : Inport  Port=3
  in4 : Inport  Port=4
  acc_len : Inport  Port=5
  Terminator : Terminator
  Terminator1 : Terminator
  Terminator2 : Terminator
  power_integrator : Subsystem
  power_integrator1 : Subsystem
  power_integrator2 : Subsystem
  power_integrator3 : Subsystem
  rst : Outport
  pow1 : Outport  Port=2
  pow2 : Outport  Port=3
  pow3 : Outport  Port=4
  pow4 : Outport  Port=5
  wires:
  acc_len/1 -> power_integrator/2(acc_len), power_integrator1/2(acc_len), power_integrator2/2(acc_len), power_integrator3/2(acc_len)
  power_integrator/2(rst_out) -> rst/1
  power_integrator1/1(pow) -> pow2/1
  power_integrator2/1(pow) -> pow3/1
  power_integrator3/1(pow) -> pow4/1
  in4/1 -> power_integrator3/1(signal)
  in3/1 -> power_integrator2/1(signal)
  in2/1 -> power_integrator1/1(signal)
  in1/1 -> power_integrator/1(signal)
  power_integrator/1(pow) -> pow1/1
  power_integrator3/2(rst_out) -> Terminator2/1
  power_integrator2/2(rst_out) -> Terminator1/1
  power_integrator1/2(rst_out) -> Terminator/1

== system read_power_16chan/power_integrator_16x/power_integrator_4x2 ==
  in1 : Inport
  in2 : Inport  Port=2
  in3 : Inport  Port=3
  in4 : Inport  Port=4
  acc_len : Inport  Port=5
  Terminator : Terminator
  Terminator1 : Terminator
  Terminator2 : Terminator
  power_integrator : Subsystem
  power_integrator1 : Subsystem
  power_integrator2 : Subsystem
  power_integrator3 : Subsystem
  rst : Outport
  pow1 : Outport  Port=2
  pow2 : Outport  Port=3
  pow3 : Outport  Port=4
  pow4 : Outport  Port=5
  wires:
  power_integrator1/2(rst_out) -> Terminator/1
  power_integrator2/2(rst_out) -> Terminator1/1
  power_integrator3/2(rst_out) -> Terminator2/1
  power_integrator/1(pow) -> pow1/1
  in1/1 -> power_integrator/1(signal)
  in2/1 -> power_integrator1/1(signal)
  in3/1 -> power_integrator2/1(signal)
  in4/1 -> power_integrator3/1(signal)
  power_integrator3/1(pow) -> pow4/1
  power_integrator2/1(pow) -> pow3/1
  power_integrator1/1(pow) -> pow2/1
  power_integrator/2(rst_out) -> rst/1
  acc_len/1 -> power_integrator3/2(acc_len), power_integrator2/2(acc_len), power_integrator1/2(acc_len), power_integrator/2(acc_len)

== system read_power_16chan/power_integrator_16x/power_integrator_4x3 ==
  in1 : Inport
  in2 : Inport  Port=2
  in3 : Inport  Port=3
  in4 : Inport  Port=4
  acc_len : Inport  Port=5
  Terminator : Terminator
  Terminator1 : Terminator
  Terminator2 : Terminator
  power_integrator : Subsystem
  power_integrator1 : Subsystem
  power_integrator2 : Subsystem
  power_integrator3 : Subsystem
  rst : Outport
  pow1 : Outport  Port=2
  pow2 : Outport  Port=3
  pow3 : Outport  Port=4
  pow4 : Outport  Port=5
  wires:
  acc_len/1 -> power_integrator/2(acc_len), power_integrator1/2(acc_len), power_integrator2/2(acc_len), power_integrator3/2(acc_len)
  power_integrator/2(rst_out) -> rst/1
  power_integrator1/1(pow) -> pow2/1
  power_integrator2/1(pow) -> pow3/1
  power_integrator3/1(pow) -> pow4/1
  in4/1 -> power_integrator3/1(signal)
  in3/1 -> power_integrator2/1(signal)
  in2/1 -> power_integrator1/1(signal)
  in1/1 -> power_integrator/1(signal)
  power_integrator/1(pow) -> pow1/1
  power_integrator3/2(rst_out) -> Terminator2/1
  power_integrator2/2(rst_out) -> Terminator1/1
  power_integrator1/2(rst_out) -> Terminator/1
